simulink model "SELECT_DETECT"  (R2024a)
settings: Solver=FixedStepAuto  StartTime=0.0  StopTime=3600  RelTol=1e-3
model workspace (MAT data in the model file):
  SampleTime = 0.001
  cameraT1_fs = 10
  cameraT2_fs = 20
  npxlsT1_syncT = 4
  senseT1_leftAmpGain = 1
  senseT1_rightAmpGain = 1
  senseT1_tactileStimRiseTime = 0.1
  senseT1_targetProbability = 0.3
  senseT1_targetSide = 1
  senseT1_triangleAmplitude = 10
  var_lick_threshold = 0.006
  var_piezo_offset = 0.0059
  var_rewardDuration = 0.03
  var_switchTime = 0
  var_trainingStage = 4
undefined symbols (not defined in the file or in its folder): Ended, Single
libraries: speedgoatlib_IO191 x5
settings Model: SimulationMode=external  ExtModeEnableFloating=off  Creator=electro  LastModifiedBy=craig
settings SolverCC: ConcurrentTasks=on  PositivePriorityOrder=on  AutoInsertRateTranBlk=on
settings DataIOCC: SaveFormat=Array
settings OptimizationCC: BlockReduction=off  OptimizeBlockIOStorage=off  EnhancedBackFolding=on  PassReuseOutputArgsThreshold=0  OptimizeBlockOrder=speed  DifferentSizesBufferReuse=on
settings DebuggingCC: TasksWithSamePriorityMsg=none  ParameterTunabilityLossMsg=error  SFUnexpectedBacktrackingDiag=warning  SFNoUnconditionalDefaultTransitionDiag=warning
settings HardwareCC: ProdBitPerLong=64  ProdLongLongMode=on  ProdHWDeviceType=Intel->x86-64 (Linux 64)
settings SFSimCC: SimUserIncludeDirs="\"/usr/local/MATLAB/R2023a/toolbox/slrealtime/target/kernel/dist/include/verify\""  MATLABDynamicMemAlloc=off
settings RTWCC: Description=Speedgoat Real-Time Target Machine  SystemTargetFile=speedgoat.tlc  TemplateMakefile=slrealtime_default_tmf  GenerateReport=on  RTWVerbose=off  CustomInclude=/usr/local/MATLAB/R2023a/toolbox/slrealtime/target/kernel/dist/include,  Toolchain=Simulink Real-Time Toolchain  BuildConfiguration=Faster Runs  CodeExecutionProfiling=on  TargetLang=C++  GPUComputeCapability=3.5
settings CodeAppCC: ForceParamTrailComments=on  OperatorAnnotations=on  EnableCustomComments=on
settings SimulinkRealTimeTargetCC: InstructionSetFMA=off  LogToMDFFile=off

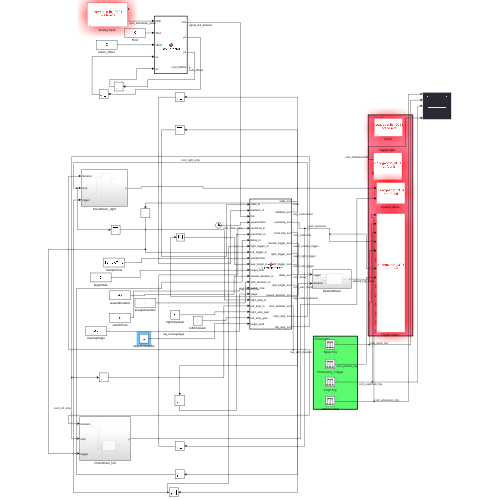
[thumbnail: Simulink's stored preview of the top-level diagram]
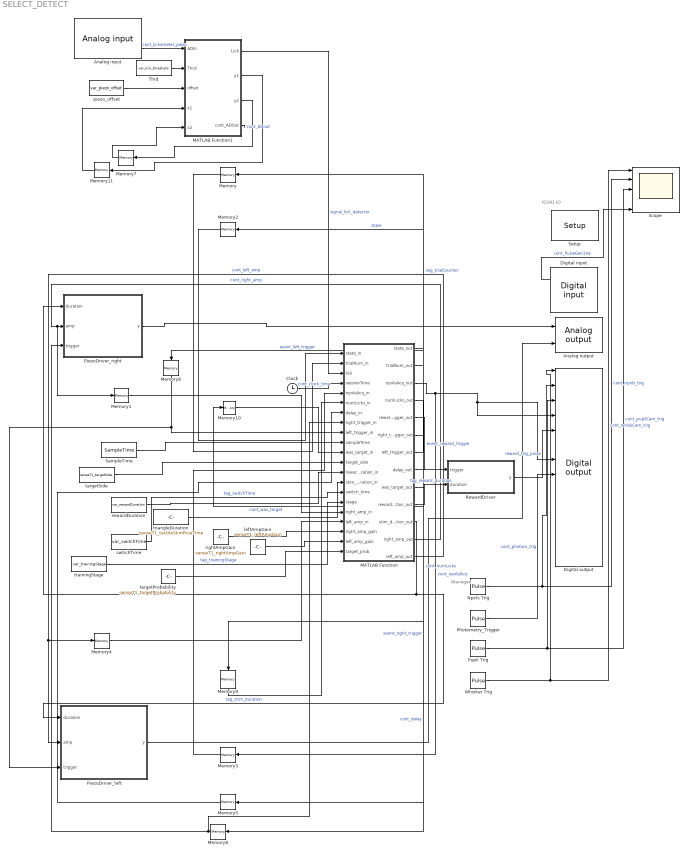
== system SELECT_DETECT ==
  note: IO191 IO
  note: Wavegen
  "Analog input " : speedgoatlib_IO191/Analog input   parModuleId=1  parSampleTime=-1  parPciSlot=-1  parAdcChannels=[1 2]  parAdcMode=2  parAdcRanges=[3 3]  parAdcInitValues=[0 0]  parAdcResets=[1 1]  paramsAdcDma=[0 1 200 -1]
      settings: SourceProductName=IO191
  "Analog output " : speedgoatlib_IO191/Analog output   parModuleId=1  parSampleTime=-1  parPciSlot=-1  parDacChannels=[1 3]  parModuleType=1  parDacRanges=[4 4]  parDacInitValues=[0 0]  parDacResets=[1 1]
      settings: SourceProductName=IO191
  Clock : Clock
      settings: Decimation=1000
  "Digital input " : speedgoatlib_IO191/Digital input   parModuleId=1  parSampleTime=SampleTime  parPciSlot=-1  parDiChannels=[9 14]
      settings: SourceProductName=IO191
  "Digital output " : speedgoatlib_IO191/Digital output   parModuleId=1  parSampleTime=0.001  parPciSlot=-1  parDoChannels=[1 2 3 4 5 6 7 8 10 11 12 13 15 16]  parDoInitValues=[0 0 0 0 0 0 0 0 0 0 0 0 0 0]  parDoResets=[1 1 1 1 1 1 1 1 1 1 1 1 1 1]
      settings: SourceProductName=IO191
  MATLAB Function : MATLAB Function  TreatAsAtomicUnit=on
  MATLAB Function1 : MATLAB Function  TreatAsAtomicUnit=on
  Memory{,1..2,4..11} (11 alike) : Memory
  Memory3 : Memory  InitialCondition=1
  Npxls Trig : DiscretePulseGenerator  Amplitude=2.5  Period=npxlsT1_syncT  PulseWidth=npxlsT1_syncT/2  SampleTime=SampleTime
  Photometry_Trigger : DiscretePulseGenerator  Amplitude=2.5  Period=npxlsT1_syncT  PulseWidth=npxlsT1_syncT/2  SampleTime=SampleTime
  PiezoDriver_left : Subsystem
  PiezoDriver_right : Subsystem
  Pupil Trig : DiscretePulseGenerator  Period=(1/cameraT1_fs) / SampleTime  PulseWidth=(1/cameraT1_fs) / SampleTime /2  SampleTime=SampleTime
  RewardDriver : Subsystem
  SampleTime : Constant  Value=SampleTime  SampleTime=SampleTime
  Scope : Scope  NumInputPorts=5
  "Setup " : speedgoatlib_IO191/Setup   parModuleId=1  parPciSlot=-1  parTriggerSignal=TTL  parAdcChannels=[1 2]  parAdcRanges=[3 3]  parAdcChannel1=on  parAdcChannel2=on  parAdcChannel3=off  parAdcChannel4=off  parAdcChannel5=off  parAdcChannel6=off  parAdcChannel7=off  parAdcChannel8=off  parAdcMode=Single-Ended  parAdcRange11=+-10.24 V  parAdcRange21=+-24.576 V  parAdcRange12=+-10.24 V  parAdcRange22=+-24.576 V  parAdcRange13=+-10.24 V  parAdcRange23=+-24.576 V  parAdcRange14=+-10.24 V  parAdcRange24=+-24.576 V  parAdcRange15=+-10.24 V  parAdcRange25=+-24.576 V  parAdcRange16=+-10.24 V  parAdcRange26=+-24.576 V  parAdcRange17=+-10.24 V  parAdcRange27=+-24.576 V  parAdcRange18=+-10.24 V  parAdcRange28=+-24.576 V  parAdcEnDma=off  parAdcFrame=125  parAdcDiv=200  parAdcSample=-1  parDacChannels=[1 3]  parDacChannel1=on  parDacChannel2=off  parDacChannel3=on  parDacChannel4=off  parDacMode=Single-Ended  parDacRanges=[4 4]  parDacInitValues=[0 0]  parDacResets=[1 1]  parDacRange1=+-10 V  parDacInitValue1=0  parDacReset1=on  parDacRange2=+-10 V  parDacInitValue2=0  parDacReset2=on  parDacRange3=+-10 V  parDacInitValue3=0  parDacReset3=on  parDacRange4=+-10 V  parDacInitValue4=0  parDacReset4=on  parDiChannels=[9 14]  parDoChannels=[1 2 3 4 5 6 7 8 10 11 12 13 15 16]  parDioFirstControl=[1 3 4 5 6 8 9]  parDioSecondControl=0  parDioChannel1=Out  parExtra1=I  parExtra2=I  parExtra3=I  parDioChannel2=In  parDioChannel3=Out  parDioChannel4=Out  parDioChannel5=Out  parDioChannel6=Out  parDioChannel7=In  parDioChannel8=Out  parDioChannel9=Out  parDoInitValues=[0 0 0 0]  parDoResets=[1 1 1 1]  parDoInitValue1=0  parDoReset1=on  parDoInitValue2=0  parDoReset2=on  parDoInitValue3=0  parDoReset3=on  parDoInitValue4=0  parDoReset4=on  parDoInitValue5=0  parDoReset5=on  parDoInitValue6=0  parDoReset6=on  parDoInitValue7=0  parDoReset7=on  parDoInitValue8=0  parDoReset8=on  parDoInitValue9=0  parDoReset9=on  parDoInitValue10=0  parDoReset10=on  parDoInitValue11=0  parDoReset11=on  parDoInitValue12=0  parDoReset12=on  parDoInitValue13=0  parDoReset13=on  parDoInitValue14=0  parDoReset14=on  parDoInitValue15=0  parDoReset15=on  parDoInitValue16=0  parDoReset16=on
      settings: SourceProductName=IO191
  Thrd : Constant  Value=var_lick_threshold
  Whisker Trig : DiscretePulseGenerator  Period=(1/cameraT2_fs) / SampleTime  PulseWidth=(1/cameraT2_fs) / SampleTime /2  SampleTime=SampleTime
  leftAmpGain : Constant  Value=senseT1_leftAmpGain
  piezo_offset : Constant  Value=var_piezo_offset
  rewardDuration : Constant  Value=var_rewardDuration
  rightAmpGain : Constant  Value=senseT1_rightAmpGain
  swtichTime : Constant  Value=var_switchTime
  targetProbability : Constant  Value=senseT1_targetProbability
  targetSide : Constant  Value=senseT1_targetSide
  trainingStage : Constant  Value=var_trainingStage
  triangleDuration : Constant  Value=senseT1_tactileStimRiseTime
  wires:
  MATLAB Function/10(reward_duration_out) -> RewardDriver/2(duration)  "tag_reward_duration"
  MATLAB Function/9(was_target_out) -> Memory10/1  "cont_was_target"
  MATLAB Function/6(right_trigger_out) -> Memory8/1  "event_right_trigger"
  MATLAB Function/4(numLicks_out) -> Memory9/1  "cont_numLicks"
  MATLAB Function/3(npxlsAcq_out) -> "Digital output "/7, "Digital output "/4, Memory3/1  "cont_npxlsAcq"
  swtichTime/1 -> MATLAB Function/15(switch_time)  "tag_switchTime"
  Thrd/1 -> MATLAB Function1/2(Thrd)
  MATLAB Function/8(delay_out) -> Memory5/1  "cont_delay"
  Memory7/1 -> MATLAB Function1/5(x2)
  "Analog input "/2 -> MATLAB Function1/1(ADIn)  "cont_lickometer_piezo"
  MATLAB Function1/2(y1) -> Memory11/1
  MATLAB Function/5(reward_trigger_out) -> RewardDriver/1(trigger)  "event_reward_trigger"
  trainingStage/1 -> MATLAB Function/16(stage)  "tag_trainingStage"
  Memory11/1 -> MATLAB Function1/4(x1)
  piezo_offset/1 -> MATLAB Function1/3(offset)
  Memory9/1 -> MATLAB Function/6(numLicks_in)
  MATLAB Function/11(stim_duration_out) -> PiezoDriver_left/1(duration), PiezoDriver_right/1(duration)  "tag_stim_duration"
  Pupil Trig/1 -> "Digital output "/3, Scope/3  "cont_pupilCam_trig"
  targetSide/1 -> MATLAB Function/12(target_side)
  MATLAB Function/7(left_trigger_out) -> Memory6/1  "event_left_trigger"
  triangleDuration/1 -> MATLAB Function/14(stim_duration_in)
  Memory8/1 -> PiezoDriver_right/3(trigger), MATLAB Function/8(right_trigger_in)
  Npxls Trig/1 -> "Digital output "/2, Scope/2  "cont_npxls_trig"
  Memory3/1 -> MATLAB Function/5(npxlsAcq_in)
  MATLAB Function1/3(y2) -> Memory7/1
  MATLAB Function/2(trialNum_out) -> Memory/1  "seg_trialCounter"
  MATLAB Function/1(state_out) -> Memory2/1  "state"
  Clock/1 -> MATLAB Function/4(sessionTime)  "cont_clock_time"
  Memory/1 -> MATLAB Function/2(trialNum_in)
  Memory2/1 -> MATLAB Function/1(state_in)
  Whisker Trig/1 -> "Digital output "/1, Scope/1  "cont_whiskCam_trig"
  Memory5/1 -> MATLAB Function/7(delay_in)
  Memory6/1 -> PiezoDriver_left/3(trigger), MATLAB Function/9(left_trigger_in)
  MATLAB Function1/1(Lick) -> MATLAB Function/3(lick)  "signal_lick_detector"
  rewardDuration/1 -> MATLAB Function/13(reward_duration_in)
  Memory10/1 -> MATLAB Function/11(was_target_in)
  SampleTime/1 -> MATLAB Function/10(sampleTime)
  RewardDriver/1(y) -> "Digital output "/5  "reward_trig_pulse"
  PiezoDriver_left/1(y) -> "Analog output "/2
  Photometry_Trigger/1 -> "Digital output "/8  "cont_photom_trig"
  PiezoDriver_right/1(y) -> "Analog output "/1
  "Digital input "/1 -> Scope/5  "cont_PulseGen1Hz"
  MATLAB Function1/4(cont_ADOut) -> ?  "cont_ADout"
  MATLAB Function/12(right_amp_out) -> Memory1/1, PiezoDriver_right/2(amp)  "cont_right_amp"
  MATLAB Function/13(left_amp_out) -> PiezoDriver_left/2(amp), Memory4/1  "cont_left_amp"
  Memory1/1 -> MATLAB Function/17(right_amp_in)
  Memory4/1 -> MATLAB Function/18(left_amp_in)
  rightAmpGain/1 -> MATLAB Function/19(right_amp_gain)
  leftAmpGain/1 -> MATLAB Function/20(left_amp_gain)
  targetProbability/1 -> MATLAB Function/21(target_prob)

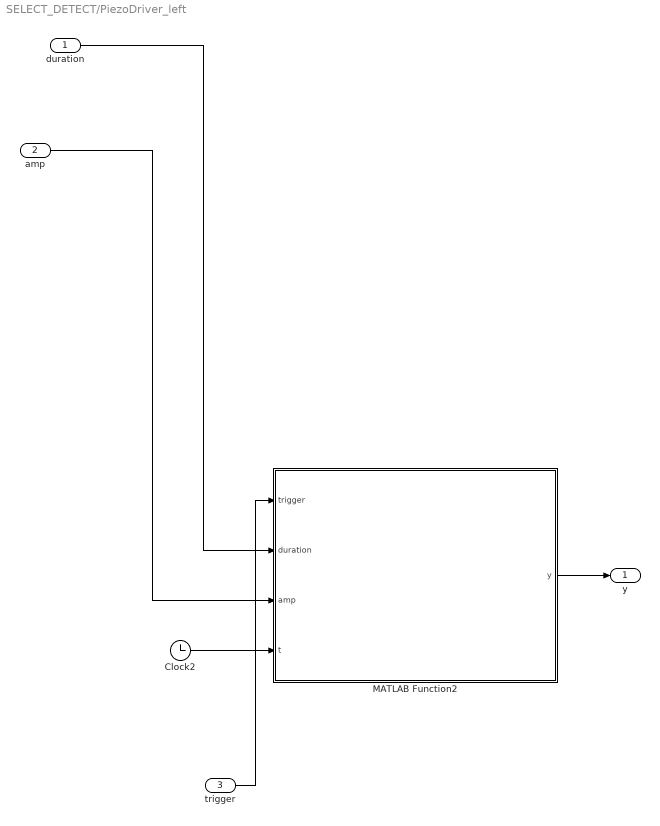
== system SELECT_DETECT/PiezoDriver_left ==
  duration : Inport
  amp : Inport  Port=2
  trigger : Inport  Port=3
  Clock2 : Clock
  MATLAB Function2 : MATLAB Function  TreatAsAtomicUnit=on
  y : Outport
  wires:
  Clock2/1 -> MATLAB Function2/4(t)
  MATLAB Function2/1(y) -> y/1
  amp/1 -> MATLAB Function2/3(amp)
  trigger/1 -> MATLAB Function2/1(trigger)
  duration/1 -> MATLAB Function2/2(duration)

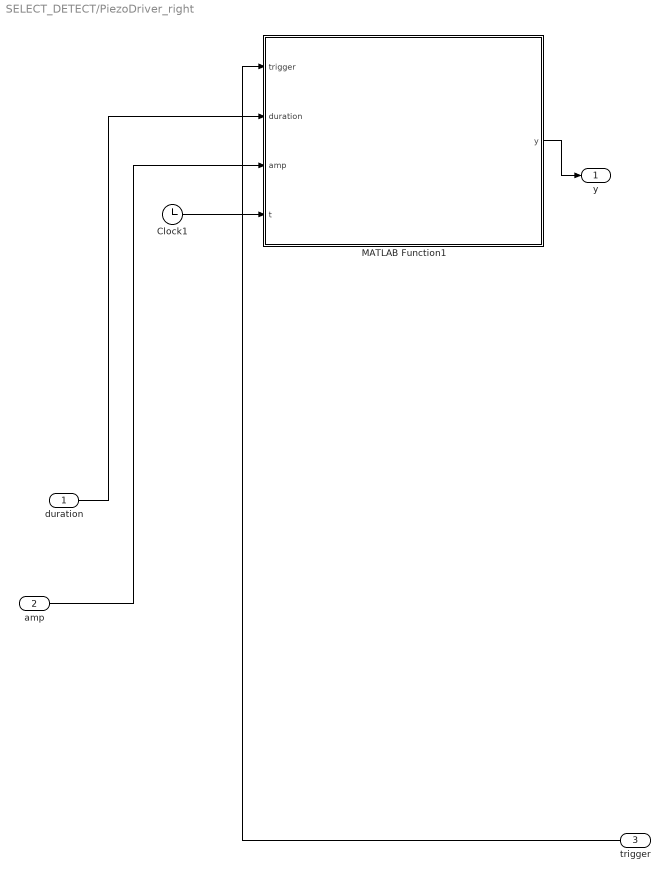
== system SELECT_DETECT/PiezoDriver_right ==
  duration : Inport
  amp : Inport  Port=2
  trigger : Inport  Port=3
  Clock1 : Clock
  MATLAB Function1 : MATLAB Function  TreatAsAtomicUnit=on
  y : Outport
  wires:
  Clock1/1 -> MATLAB Function1/4(t)
  trigger/1 -> MATLAB Function1/1(trigger)
  amp/1 -> MATLAB Function1/3(amp)
  duration/1 -> MATLAB Function1/2(duration)
  MATLAB Function1/1(y) -> y/1

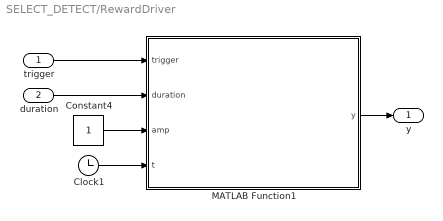
== system SELECT_DETECT/RewardDriver ==
  trigger : Inport
  duration : Inport  Port=2
  Clock1 : Clock
  Constant4 : Constant  SampleTime=SampleTime
  MATLAB Function1 : MATLAB Function  TreatAsAtomicUnit=on
  y : Outport
  wires:
  Clock1/1 -> MATLAB Function1/4(t)
  Constant4/1 -> MATLAB Function1/3(amp)
  duration/1 -> MATLAB Function1/2(duration)
  trigger/1 -> MATLAB Function1/1(trigger)
  MATLAB Function1/1(y) -> y/1

== matlab function SELECT_DETECT/PiezoDriver_right/MATLAB Function1 ==
  data: trigger input; duration input; amp input; y output; t input
function y = drivePiezo(trigger, duration, amp, t) 
    % When the trigger is received, drivePiezo starts to output a triangle 
    % wave defined by duration and amplitude
    
    % If the trigger is not received, it checks whether t0 is not 
    % empty (indicating that a trigger has been received previously). 
    % If t0 is not empty, it checks if (t - t0) is less than 1.5 seconds. 
    % If so, it keeps tonePulse set to 1, maintaining the tone pulse for 
    % 1.5 seconds after the trigger. 
      
    
    persistent t0;
    persistent y0;
    increment = amp / (duration*1000/2);

    if trigger                
        t0 = t; % store current time 
        y = 0;
        y0 = y;
    elseif ~isempty(t0) 
        if (t - t0) <= duration/2
            y = y0 + increment;
            y0 = y;
        elseif (t - t0) <= duration
            y = y0 - increment;
            y = max([0,y]);
            y0 = y;
        else
            y = 0;
            clear t0 y0 % reset t0 to initial condition
        end        
    else % reset to 0 if no more trigger activity
        y = 0;        
    end

end

== matlab function SELECT_DETECT/RewardDriver/MATLAB Function1 ==
  data: trigger input; y output; duration input; amp input; t input
function y = driveSpout(trigger, duration, amp, t) 
    % When the trigger is received, driveSpout starts to output a square
    % pulse defined by duration and amplitude
    
    % If the trigger is not received, it checks whether t0 is not 
    % empty (indicating that a trigger has been received previously). 
    % If t0 is not empty, it checks if (t - t0) is less than 1.5 seconds. 
    % If so, it keeps tonePulse set to 1, maintaining the tone pulse for 
    % 1.5 seconds after the trigger. 
      
    
    persistent t0;

    if trigger                     
        t0 = t; % store current time 
        y = amp;
    elseif ~isempty(t0) 
        if (t - t0) <= duration
            y = amp;
        else
            y = 0;
            clear t0 % reset t0 to initial condition
        end        
    else % reset to 0 if no more trigger activity
        y = 0;        
    end
end

== matlab function SELECT_DETECT/MATLAB Function1 ==
  data: ADIn input; Lick output; y1 output; Thrd input; offset input; x1 input; x2 input; y2 output; cont_ADOut output
function [Lick, y1, y2, cont_ADOut] = LickDetector(ADIn, Thrd, offset, x1, x2)

    [Lick, y1, y2, cont_ADOut] = detectLicks(ADIn, Thrd, offset, x1, x2);

end

== matlab function SELECT_DETECT/MATLAB Function ==
  data: state_in input; trialNum_in input; lick input; sessionTime input; npxlsAcq_in input; state_out output; trialNum_out output; npxlsAcq_out output; numLicks_in input; delay_in input; right_trigger_in input; left_trigger_in input; sampleTime input; numLicks_out output; reward_trigger_out output; right_trigger_out output; left_trigger_out output; delay_out output; was_target_in input; was_target_out output; target_side input; reward_duration_in input; stim_duration_in input; switch_time input; stage input; reward_duration_out output; stim_duration_out output; right_amp_out output; left_amp_out output; right_amp_in input; left_amp_in input; right_amp_gain input; left_amp_gain input; target_prob input
function [state_out, trialNum_out, ...
    npxlsAcq_out, numLicks_out, reward_trigger_out, ...
    right_trigger_out, left_trigger_out, delay_out, was_target_out, ... 
    reward_duration_out, stim_duration_out, right_amp_out, left_amp_out] ...
    = SELECT_DETECT(state_in, trialNum_in, lick, ...
    sessionTime, npxlsAcq_in, numLicks_in, delay_in, ... 
    right_trigger_in, left_trigger_in, sampleTime, was_target_in, ...
    target_side, reward_duration_in, stim_duration_in, switch_time, stage, ...
    right_amp_in, left_amp_in, right_amp_gain, left_amp_gain, target_prob)

    % stages: 1 - classical conditioning, 2 - opreant conditioning, 3 - impulse
    % control, 111 - calibrate reward delivery; 222 - position piezo; 333 -
    % calibrate piezo driver triangle duration 
    
    [state_out, trialNum_out, ...
    npxlsAcq_out, numLicks_out, reward_trigger_out, ...
    right_trigger_out, left_trigger_out, delay_out, was_target_out, ... 
    reward_duration_out, stim_duration_out, right_amp_out, left_amp_out] ...
    = behavior_control(state_in, trialNum_in, lick, ...
    sessionTime, npxlsAcq_in, numLicks_in, delay_in, ... 
    right_trigger_in, left_trigger_in, sampleTime, was_target_in, ...
    target_side, reward_duration_in, stim_duration_in, switch_time, stage, ...
    right_amp_in, left_amp_in, right_amp_gain, left_amp_gain, target_prob);

end

== matlab function SELECT_DETECT/PiezoDriver_left/MATLAB Function2 ==
  data: trigger input; duration input; amp input; y output; t input
function y = drivePiezo(trigger, duration, amp, t) 
    % When the trigger is received, drivePiezo starts to output a triangle 
    % wave defined by duration and amplitude
    
    % If the trigger is not received, it checks whether t0 is not 
    % empty (indicating that a trigger has been received previously). 
    % If t0 is not empty, it checks if (t - t0) is less than 1.5 seconds. 
    % If so, it keeps tonePulse set to 1, maintaining the tone pulse for 
    % 1.5 seconds after the trigger. 
      
    
    persistent t0;
    persistent y0;
    increment = amp / (duration*1000/2);

    if trigger                
        t0 = t; % store current time 
        y = 0;
        y0 = y;
    elseif ~isempty(t0) 
        if (t - t0) <= duration/2
            y = y0 + increment;
            y0 = y;
        elseif (t - t0) <= duration
            y = y0 - increment;
            y = max([0,y]);
            y0 = y;
        else
            y = 0;
            clear t0 y0 % reset t0 to initial condition
        end        
    else % reset to 0 if no more trigger activity
        y = 0;        
    end

end
